simulink model "2xDAC"  (R2016b)
settings: Solver=FixedStepDiscrete  StartTime=0.0  StopTime=10.0  FixedStep=1e-3  RelTol=1e-3
libraries: mbed_lib x7
settings Model: Creator=oh  LastModifiedBy=oh
settings OptimizationCC: DefaultParameterBehavior=Inlined
settings DebuggingCC: ParameterTunabilityLossMsg=error
settings HardwareCC: ProdBitPerPointer=32  ProdBitPerSizeT=32  ProdBitPerPtrDiffT=32  ProdLargestAtomicInteger=Long  ProdLargestAtomicFloat=Double  ProdWordSize=32  ProdHWDeviceType=ARM Compatible->ARM Cortex
settings RTWCC: SystemTargetFile=mbed.tlc  TemplateMakefile=mbed.tmf  Description=Mbed Target (Embedded Target)  GenerateReport=on  IncludeHyperlinkInReport=on  TargetLang=C++  GenerateTraceInfo=on  GenerateTraceReport=on  GenerateTraceReportSl=on  GenerateTraceReportSf=on  GenerateTraceReportEml=on
settings CodeAppCC: ForceParamTrailComments=on  IgnoreCustomStorageClasses=off  OperatorAnnotations=on  SimulinkDataObjDesc=on  SFDataObjDesc=on  MATLABFcnDesc=on  InsertBlockDesc=on  MATLABSourceComments=on
settings STFCustomTargetCC: TargetLibSuffix=.a  TargetLangStandard=C++03 (ISO)  GenerateSampleERTMain=on  CombineOutputUpdateFcns=on  ERTCustomFileBanners=on  SupportContinuousTime=off  SupportNonInlinedSFcns=off  RemoveResetFunc=on  MATLABClassNameForMDSCustomization=Simulink.SoftwareTarget.ERTCustomization  GRTInterface=off  SystemTargetFile=mbed.tlc
settings ERTTargetCC: TargetLangStandard=C++03 (ISO)  GenerateSampleERTMain=on  ParMdlRefBuildCompliant=off  CompOptLevelCompliant=off  ConcurrentExecutionCompliant=off  ERTFirstTimeCompliant=off  ModelStepFunctionPrototypeControlCompliant=off  CPPClassGenCompliant=off  UseToolchainInfoCompliant=off  InlinedParameterPlacement=NonHierarchical  ERTCustomFileTemplate=mbed_file_process.tlc

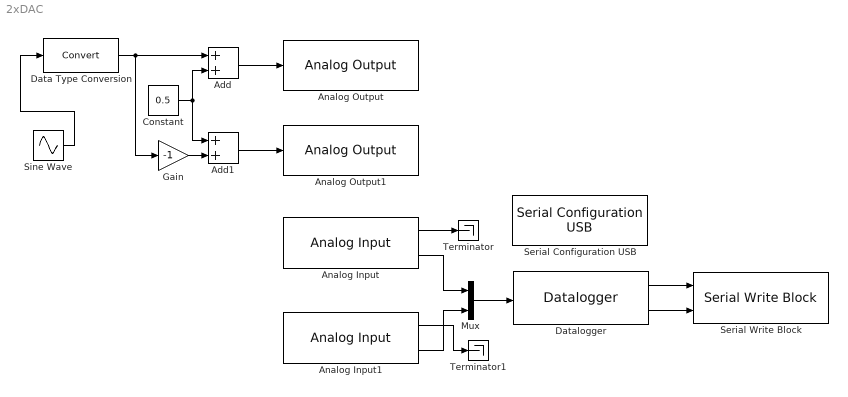
== system 2xDAC ==
  Add : Sum
  Add1 : Sum
  Analog Input : mbed_lib/GPIO/Analog Input  PortName=A  PinNumber=3  SampleTime=0.05
  Analog Input1 : mbed_lib/GPIO/Analog Input  PortName=A  PinNumber=6  SampleTime=0.05
  Analog Output : mbed_lib/GPIO/Analog Output  PortName=A  PinNumber=4  Mode=Double: 0 - 1.0f  SampleTime=-1
  Analog Output1 : mbed_lib/GPIO/Analog Output  PortName=A  PinNumber=5  Mode=Double: 0 - 1.0f  SampleTime=-1
  Constant : Constant  Value=0.5  OutDataTypeStr=single
  Data Type Conversion : DataTypeConversion
  Datalogger : mbed_lib/Utilities/Datalogger  TypeInputPorts={ 'single' 2 }  TypeOfInputs={'2*single'}  BufferSize=100  errEn=off  SampleTime=-1
  Gain : Gain  Gain=-1
  Mux : Mux  Inputs=2
  Serial Configuration USB : mbed_lib/Serial/UART/Serial Configuration USB  BaudRate=115200
  Serial Write Block : mbed_lib/Serial/UART/Serial Write Block  SerialPort=0  numData=on  SampleTime=-1
  Sine Wave : Sin  Amplitude=0.5  Frequency=10  SampleTime=0.01
  Terminator : Terminator
  Terminator1 : Terminator
  wires:
  Sine Wave/1 -> Data Type Conversion/1
  Mux/1 -> Datalogger/1
  Analog Input/2 -> Mux/1
  Analog Input1/2 -> Mux/2
  Datalogger/1 -> Serial Write Block/1
  Datalogger/2 -> Serial Write Block/2
  Analog Input/1 -> Terminator/1
  Analog Input1/1 -> Terminator1/1
  Data Type Conversion/1 -> Add/1, Gain/1
  Add/1 -> Analog Output/1
  Gain/1 -> Add1/2
  Add1/1 -> Analog Output1/1
  Constant/1 -> Add/2, Add1/1
